simulink model "sensorFusionTask"  (R2015b)
settings: Solver=FixedStepDiscrete  StartTime=0.0  StopTime=inf  FixedStep=1/1000  RelTol=1e-3
libraries: simulink x3, embdlinuxlib x1
settings Model: SimulationMode=external  ExtModeEnableFloating=off  ExtModeTrigDuration=100  Creator=Nik Descher  LastModifiedBy=Nik Descher
settings DataIOCC: LimitDataPoints=off
settings OptimizationCC: OptimizeModelRefInitCode=on  LifeSpan=1
settings HardwareCC: ProdBitPerPointer=32  ProdLargestAtomicInteger=Long  ProdLargestAtomicFloat=Double  ProdWordSize=32  ProdHWDeviceType=ARM Compatible->ARM Cortex
settings RTWCC: SystemTargetFile=realtime.tlc  GenerateMakefile=off  TemplateMakefile=realtime.tmf  Description=Run on Target Hardware  RTWVerbose=off
settings STFCustomTargetCC: TargetLibSuffix=.a  GenerateSampleERTMain=on  ConcurrentExecutionCompliant=off  GeneratePreprocessorConditionals=Use local settings  ERTCustomFileBanners=on  SupportNonInlinedSFcns=off  SupportVariableSizeSignals=on  MATLABClassNameForMDSCustomization=Simulink.SoftwareTarget.ERTCustomization  CPPClassGenCompliant=off  GRTInterface=off  SystemTargetFile=realtime.tlc
settings ERTTargetCC: GenerateSampleERTMain=on  ParMdlRefBuildCompliant=off  CompOptLevelCompliant=off  ConcurrentExecutionCompliant=off  CombineOutputUpdateFcns=off  ERTFirstTimeCompliant=off  SupportContinuousTime=on  SupportVariableSizeSignals=on  ModelStepFunctionPrototypeControlCompliant=off  CPPClassGenCompliant=off  UseToolchainInfoCompliant=off  ExtModeMexArgs='192.168.1.248' 0 17724  ERTSrcFileBannerTemplate=realtime_code_template.cgt  ERTHdrFileBannerTemplate=realtime_code_template.cgt  ERTDataSrcFileTemplate=realtime_code_template.cgt  ERTDataHdrFileTemplate=realtime_code_template.cgt  ERTCustomFileTemplate=realtime_file_process.tlc

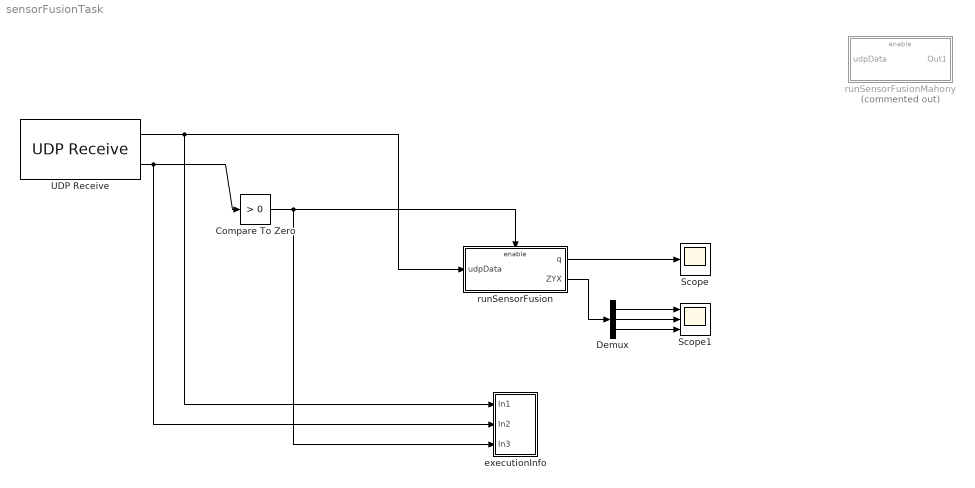
== system sensorFusionTask ==
  Compare To Zero : simulink/Logic and Bit Operations/Compare To Zero  relop=>  OutDataTypeStr=boolean
  Demux : Demux  Outputs=3
  Scope : Scope
  Scope1 : Scope  NumInputPorts=3
  UDP Receive : embdlinuxlib/UDP Receive  localURL='0.0.0.0'  localPort=25000  remoteURL='0.0.0.0'  remotePort=-1  recvBufferSize=8192  signalDatatype=single  dims=31  isVarSize=off  showBlockingTime=off  blockingTime=0  sampletime=1/1000  blockPlatform=Raspberry Pi
  executionInfo : Subsystem
  runSensorFusion : Subsystem  TreatAsAtomicUnit=on
  runSensorFusionMahony : Subsystem  Commented=on  TreatAsAtomicUnit=on
  wires:
  UDP Receive/1 -> executionInfo/1(In1), runSensorFusion/1(udpData)
  UDP Receive/2 -> executionInfo/2(In2), Compare To Zero/1
  Compare To Zero/1 -> executionInfo/3(In3), runSensorFusion/Enable
  runSensorFusion/1(q) -> Scope/1
  Demux/1 -> Scope1/1
  Demux/2 -> Scope1/2
  Demux/3 -> Scope1/3
  runSensorFusion/2(ZYX) -> Demux/1

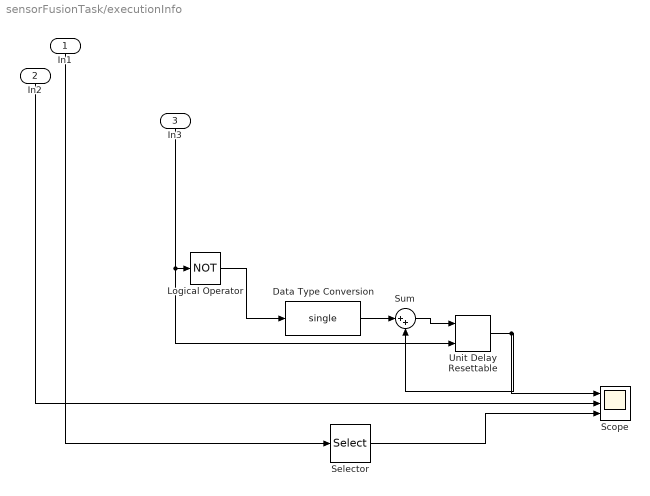
== system sensorFusionTask/executionInfo ==
  In1 : Inport
  In2 : Inport  Port=2
  In3 : Inport  Port=3
  Data Type Conversion : DataTypeConversion  OutDataTypeStr=single
  Logical Operator : Logic  Operator=NOT  AllPortsSameDT=off  OutDataTypeStr=boolean
  Scope : Scope  NumInputPorts=3
  Selector : Selector  InputPortWidth=31  IndexOptions=Index vector (dialog)  Indices=31  OutputSizes=1
  Sum : Sum  Inputs=|++
  Unit Delay Resettable : simulink/Additional Math & Discrete/Additional Discrete/Unit Delay Resettable  vinit=0  tsamp=-1
  wires:
  Unit Delay Resettable/1 -> Scope/1, Sum/2
  Data Type Conversion/1 -> Sum/1
  Sum/1 -> Unit Delay Resettable/1
  Logical Operator/1 -> Data Type Conversion/1
  Selector/1 -> Scope/3
  In3/1 -> Unit Delay Resettable/2, Logical Operator/1
  In1/1 -> Selector/1
  In2/1 -> Scope/2

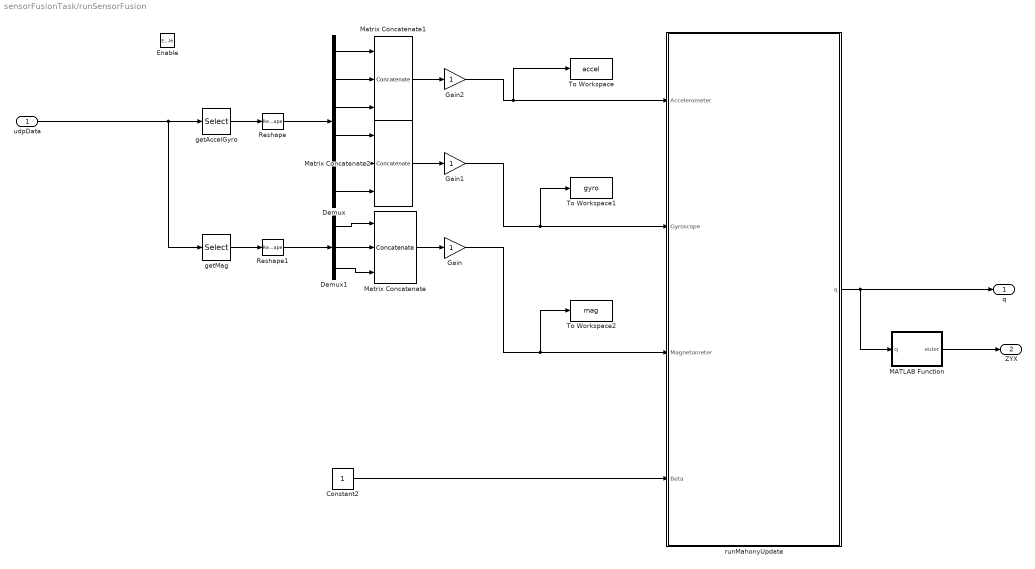
== system sensorFusionTask/runSensorFusion ==
  udpData : Inport
  Enable : EnablePort
  Constant2 : Constant  OutDataTypeStr=single
  Demux : Demux  Outputs=6
  Demux1 : Demux  Outputs=3
  Gain : Gain
  Gain1 : Gain
  Gain2 : Gain
  MATLAB Function : MATLAB Function  TreatAsAtomicUnit=on
  Matrix Concatenate : Concatenate  NumInputs=3  Mode=Multidimensional array
  Matrix Concatenate1 : Concatenate  NumInputs=3  Mode=Multidimensional array
  Matrix Concatenate2 : Concatenate  NumInputs=3  Mode=Multidimensional array
  Reshape : Reshape
  Reshape1 : Reshape
  To Workspace : ToWorkspace  VariableName=accel  SaveFormat=Structure With Time  SampleTime=-1
  To Workspace1 : ToWorkspace  VariableName=gyro  SaveFormat=Structure With Time  SampleTime=-1
  To Workspace2 : ToWorkspace  VariableName=mag  SaveFormat=Structure With Time  SampleTime=-1
  getAccelGyro : Selector  InputPortWidth=31  IndexOptions=Index vector (dialog)  Indices=1:24  OutputSizes=1
  getMag : Selector  InputPortWidth=31  IndexOptions=Index vector (dialog)  Indices=25:30  OutputSizes=1
  runMahonyUpdate : MATLAB Function  TreatAsAtomicUnit=on
  q : Outport
  ZYX : Outport  Port=2
  wires:
  getAccelGyro/1 -> Reshape/1
  Reshape/1 -> Demux/1
  Reshape1/1 -> Demux1/1
  udpData/1 -> getMag/1, getAccelGyro/1
  getMag/1 -> Reshape1/1
  Demux1/2 -> Matrix Concatenate/2
  Demux1/1 -> Matrix Concatenate/1
  Demux1/3 -> Matrix Concatenate/3
  Demux/2 -> Matrix Concatenate1/2
  Demux/3 -> Matrix Concatenate1/3
  Demux/1 -> Matrix Concatenate1/1
  Demux/4 -> Matrix Concatenate2/1
  Demux/5 -> Matrix Concatenate2/2
  Demux/6 -> Matrix Concatenate2/3
  Matrix Concatenate1/1 -> Gain2/1
  Matrix Concatenate2/1 -> Gain1/1
  Matrix Concatenate/1 -> Gain/1
  Constant2/1 -> runMahonyUpdate/4(Beta)
  runMahonyUpdate/1(q) -> MATLAB Function/1(q), q/1
  Gain/1 -> To Workspace2/1, runMahonyUpdate/3(Magnetometer)
  Gain1/1 -> To Workspace1/1, runMahonyUpdate/2(Gyroscope)
  Gain2/1 -> To Workspace/1, runMahonyUpdate/1(Accelerometer)
  MATLAB Function/1(euler) -> ZYX/1

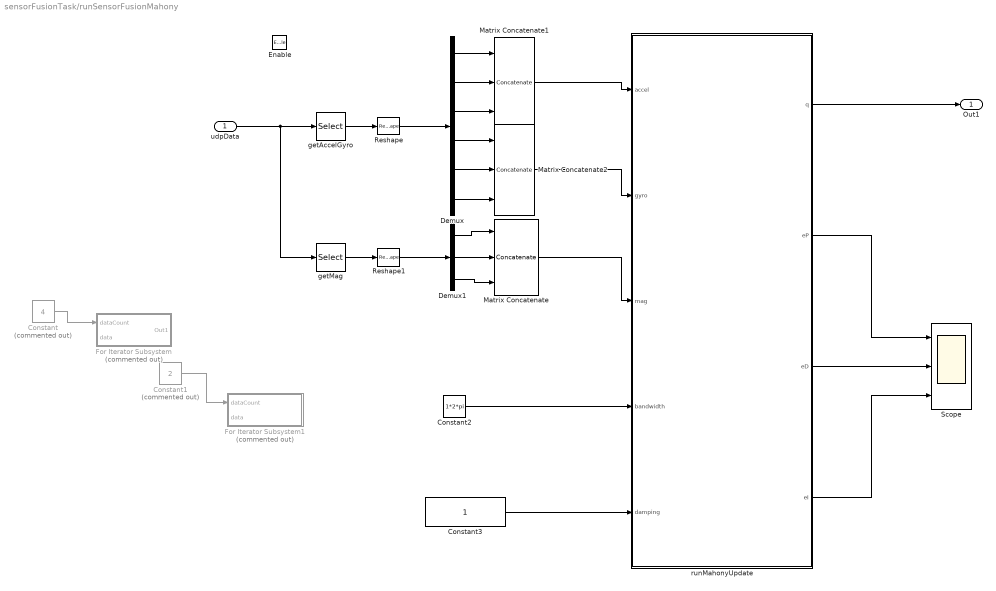
== system sensorFusionTask/runSensorFusionMahony ==
  udpData : Inport
  Enable : EnablePort
  Constant : Constant  Commented=on  Value=4
  Constant1 : Constant  Commented=on  Value=2
  Constant2 : Constant  Value=1*2*pi  OutDataTypeStr=single
  Constant3 : Constant  OutDataTypeStr=single
  Demux : Demux  Outputs=6
  Demux1 : Demux  Outputs=3
  For Iterator Subsystem : Subsystem  Commented=on  TreatAsAtomicUnit=on
  For Iterator Subsystem1 : Subsystem  Commented=on  TreatAsAtomicUnit=on
  Matrix Concatenate : Concatenate  NumInputs=3  Mode=Multidimensional array
  Matrix Concatenate1 : Concatenate  NumInputs=3  Mode=Multidimensional array
  Matrix Concatenate2 : Concatenate  NumInputs=3  Mode=Multidimensional array
  Reshape : Reshape
  Reshape1 : Reshape
  Scope : Scope  NumInputPorts=3
  getAccelGyro : Selector  InputPortWidth=31  IndexOptions=Index vector (dialog)  Indices=1:24  OutputSizes=1
  getMag : Selector  InputPortWidth=31  IndexOptions=Index vector (dialog)  Indices=25:30  OutputSizes=1
  runMahonyUpdate : MATLAB Function  TreatAsAtomicUnit=on
  Out1 : Outport
  wires:
  runMahonyUpdate/4(eI) -> Scope/3
  runMahonyUpdate/3(eD) -> Scope/2
  runMahonyUpdate/2(eP) -> Scope/1
  runMahonyUpdate/1(q) -> Out1/1
  Constant3/1 -> runMahonyUpdate/5(damping)
  Constant2/1 -> runMahonyUpdate/4(bandwidth)
  Matrix Concatenate/1 -> runMahonyUpdate/3(mag)
  Matrix Concatenate2/1 -> runMahonyUpdate/2(gyro)
  Matrix Concatenate1/1 -> runMahonyUpdate/1(accel)
  Demux/6 -> Matrix Concatenate2/3
  Demux/5 -> Matrix Concatenate2/2
  Demux/4 -> Matrix Concatenate2/1
  Demux/1 -> Matrix Concatenate1/1
  Demux/3 -> Matrix Concatenate1/3
  Demux/2 -> Matrix Concatenate1/2
  Demux1/3 -> Matrix Concatenate/3
  Demux1/1 -> Matrix Concatenate/1
  Demux1/2 -> Matrix Concatenate/2
  getMag/1 -> Reshape1/1
  udpData/1 -> getAccelGyro/1, getMag/1
  Reshape1/1 -> Demux1/1
  Reshape/1 -> Demux/1
  getAccelGyro/1 -> Reshape/1
  Constant1/1 -> For Iterator Subsystem1/1(dataCount)
  Constant/1 -> For Iterator Subsystem/1(dataCount)

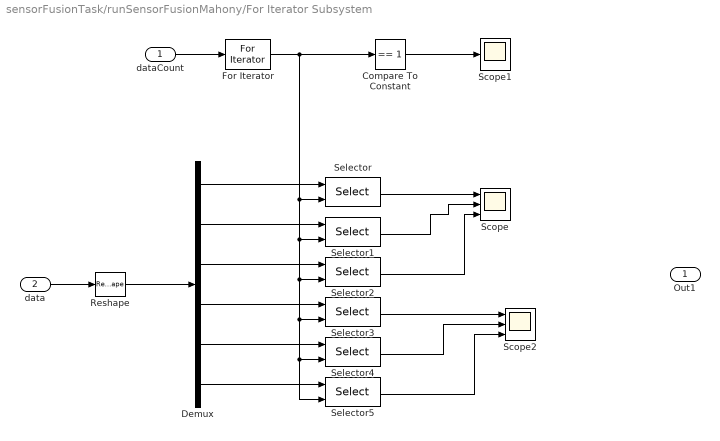
== system sensorFusionTask/runSensorFusionMahony/For Iterator Subsystem ==
  dataCount : Inport
  data : Inport  Port=2
  Compare To Constant : simulink/Logic and Bit Operations/Compare To Constant  relop===  const=1  OutDataTypeStr=boolean
  Demux : Demux  Outputs=6
  For Iterator : ForIterator  IterationSource=external
  Reshape : Reshape
  Scope : Scope  NumInputPorts=3
  Scope1 : Scope
  Scope2 : Scope  NumInputPorts=3
  Selector{,1..5} (6 alike) : Selector  InputPortWidth=4  IndexOptions=Index vector (port)  Indices=[1 3]  OutputSizes=1
  Out1 : Outport
  wires:
  Selector5/1 -> Scope2/3
  Selector4/1 -> Scope2/2
  Selector3/1 -> Scope2/1
  Reshape/1 -> Demux/1
  Compare To Constant/1 -> Scope1/1
  Selector2/1 -> Scope/3
  Selector1/1 -> Scope/2
  Selector/1 -> Scope/1
  Demux/6 -> Selector5/1
  Demux/5 -> Selector4/1
  Demux/4 -> Selector3/1
  Demux/3 -> Selector2/1
  Demux/2 -> Selector1/1
  For Iterator/1 -> Selector/2, Selector1/2, Selector2/2, Selector3/2, Selector4/2, Selector5/2, Compare To Constant/1
  Demux/1 -> Selector/1
  data/1 -> Reshape/1
  dataCount/1 -> For Iterator/1

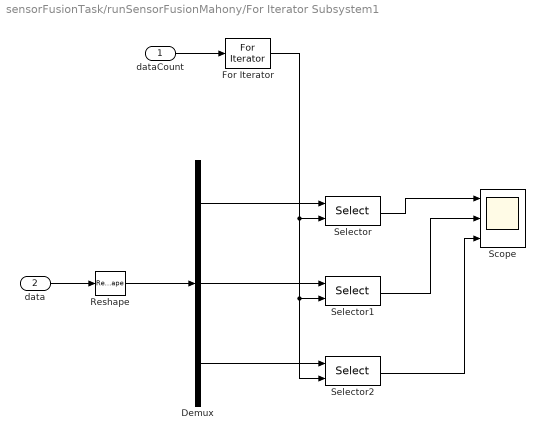
== system sensorFusionTask/runSensorFusionMahony/For Iterator Subsystem1 ==
  dataCount : Inport
  data : Inport  Port=2
  Demux : Demux  Outputs=3
  For Iterator : ForIterator  IterationSource=external
  Reshape : Reshape
  Scope : Scope  NumInputPorts=3
  Selector : Selector  InputPortWidth=2  IndexOptions=Index vector (port)  Indices=[1 3]  OutputSizes=1
  Selector1 : Selector  InputPortWidth=2  IndexOptions=Index vector (port)  Indices=[1 3]  OutputSizes=1
  Selector2 : Selector  InputPortWidth=2  IndexOptions=Index vector (port)  Indices=[1 3]  OutputSizes=1
  wires:
  dataCount/1 -> For Iterator/1
  data/1 -> Reshape/1
  Demux/1 -> Selector/1
  For Iterator/1 -> Selector2/2, Selector1/2, Selector/2
  Demux/2 -> Selector1/1
  Demux/3 -> Selector2/1
  Selector/1 -> Scope/1
  Selector1/1 -> Scope/2
  Selector2/1 -> Scope/3
  Reshape/1 -> Demux/1

== matlab function sensorFusionTask/runSensorFusionMahony/runMahonyUpdate ==
  data: accel input single size=[3 4]; q output; gyro input single size=[3 4]; mag input single size=[3 2]; bandwidth input; damping input; eP output; eD output; eI output
function [q,eP,eD,eI] = runMahonyUpdate(accel,gyro,mag,bandwidth,damping)
persistent qLocal
if isempty(qLocal)
    qLocal=single([ 1 0 0 0]);
end

magInterp=interp1([1 4],mag',[1 2 3 4],'linear')';

for i=1:4
    [qLocal,eP,eD,eI]=UpdateMahony(qLocal,gyro(:,i),accel(:,i),magInterp(:,i),bandwidth,damping);
end

q=qLocal;



 function [q,eP,eD,eI] = UpdateMahony(q,Gyroscope, Accelerometer, Magnetometer,bandwidth,damping)
     persistent eInt eLast
     if isempty(eInt)
         eInt=single([0; 0; 0]);
     end
     if abs(bandwidth)<1e-4 && abs(damping)<1e-4
         q=single([1 0 0 0]);
         eP=single([0;0;0]);
         eD=eP;
         eI=eP;
         return;
     end
%      bandwidth = (1*2*pi);
%      damping=1;
     Ki=bandwidth^2*bandwidth;
     Kp=bandwidth^2+2*damping*bandwidth*bandwidth;
     Kd=2*damping*bandwidth+bandwidth;
% 
%      Ki=0;
%      Kp=1;
%      Kd=0;
     
     SamplePeriod=5/1000;
     % Normalise accelerometer measurement
%      if(norm(Accelerometer) == 0), return; end   % handle NaN
     Accelerometer = Accelerometer / norm(Accelerometer);    % normalise magnitude
     
     % Normalise magnetometer measurement
%      if(norm(Magnetometer) == 0), return; end    % handle NaN
     Magnetometer = Magnetometer / norm(Magnetometer);   % normalise magnitude
     
     % Reference direction of Earth's magnetic feild
     h = quaternProd(q, quaternProd([0; Magnetometer], quaternConj(q)));
     b = [0; norm([h(2); h(3)]); 0; h(4)];
     
     % Estimated direction of gravity and magnetic field
     v = [2*(q(2)*q(4) - q(1)*q(3))
         2*(q(1)*q(2) + q(3)*q(4))
         q(1)^2 - q(2)^2 - q(3)^2 + q(4)^2];
     w = [2*b(2)*(0.5 - q(3)^2 - q(4)^2) + 2*b(4)*(q(2)*q(4) - q(1)*q(3))
         2*b(2)*(q(2)*q(3) - q(1)*q(4)) + 2*b(4)*(q(1)*q(2) + q(3)*q(4))
         2*b(2)*(q(1)*q(3) + q(2)*q(4)) + 2*b(4)*(0.5 - q(2)^2 - q(3)^2)];
     
     % Error is sum of cross product between estimated direction and measured direction of fields
     e = cross(Accelerometer, v) + cross(Magnetometer, w);
     if(Ki > 0)
         eInt = eInt + e * SamplePeriod;
     else
         eInt = single([0; 0; 0]);
     end
     if isempty(eLast)
         eLast=e;
     end
     
     % Apply feedback terms
     eP=e;
     eD=e-eLast;
     eI=eInt;
     Gyroscope = Gyroscope + Kp * eP + Ki * eInt + Kd * (eD) / SamplePeriod;
     eLast=e;
     
     % Compute rate of change of quaternion
     qDot = 0.5 * quaternProd(q, [0 Gyroscope(1) Gyroscope(2) Gyroscope(3)]);
     
     % Integrate to yield quaternion
     q = q + qDot * SamplePeriod;
     q = q / norm(q); % normalise quaternion
     

function ab = quaternProd(a, b)
    ab=zeros(1,4);
%QUATERNPROD Calculates the quaternion product
%
%   ab = quaternProd(a, b)
%
%   Calculates the quaternion product of quaternion a and b.
%
%   For more information see:
%   http://www.x-io.co.uk/node/8#quaternions
%
%	Date          Author          Notes
%	27/09/2011    SOH Madgwick    Initial release

    ab(1) = a(1).*b(1)-a(2).*b(2)-a(3).*b(3)-a(4).*b(4);
    ab(2) = a(1).*b(2)+a(2).*b(1)+a(3).*b(4)-a(4).*b(3);
    ab(3) = a(1).*b(3)-a(2).*b(4)+a(3).*b(1)+a(4).*b(2);
    ab(4) = a(1).*b(4)+a(2).*b(3)-a(3).*b(2)+a(4).*b(1);

function qConj = quaternConj(q)
%QUATERN2ROTMAT Converts a quaternion to its conjugate
%
%   qConj = quaternConj(q)
%
%   Converts a quaternion to its conjugate.
%
%   For more information see:
%   http://www.x-io.co.uk/node/8#quaternions
%
%	Date          Author          Notes
%	27/09/2011    SOH Madgwick    Initial release

    qConj = [q(1) -q(2) -q(3) -q(4)];

== matlab function sensorFusionTask/runSensorFusion/runMahonyUpdate ==
  data: Accelerometer input single size=[3 4]; q output single size=[1 4]; Gyroscope input single size=[3 4]; Magnetometer input single size=[3 2]; Beta input single size=1
function q  = runMadwickUpdates(Accelerometer,Gyroscope,Magnetometer,Beta)
persistent qLocal
if isempty(qLocal)
    qLocal=single([1 0 0 0]);
end
qIn=qLocal;

magInterp=interp1([1 4],Magnetometer',[1 2 3 4],'linear')';

for i=1:4
    
    q  = runMadwickUpdate(qIn,Accelerometer(:,i),Gyroscope(:,i),magInterp(:,i),Beta);
    qIn = q;
    
end

qLocal=q;

function q  = runMadwickUpdate(qIn,Accelerometer,Gyroscope,Magnetometer,Beta)
q=qIn;
SamplePeriod=single(5/1000);

% Normalise accelerometer measurement
if ~all(abs(Accelerometer)<.0001);
    Accelerometer = Accelerometer / norm(Accelerometer);	% normalise magnitude
end
% Normalise magnetometer measurement
if ~all(abs(Magnetometer)<.0001)
    Magnetometer = Magnetometer / norm(Magnetometer);	% normalise magnitude
end
% Reference direction of Earth's magnetic feild
h = quaternProd(q, quaternProd([0 Magnetometer'], quaternConj(q)));
b = [0 norm([h(2) h(3)]) 0 h(4)];
% Gradient decent algorithm corrective step
F = [2*(q(2)*q(4) - q(1)*q(3)) - Accelerometer(1)
    2*(q(1)*q(2) + q(3)*q(4)) - Accelerometer(2)
    2*(0.5 - q(2)^2 - q(3)^2) - Accelerometer(3)
    2*b(2)*(0.5 - q(3)^2 - q(4)^2) + 2*b(4)*(q(2)*q(4) - q(1)*q(3)) - Magnetometer(1)
    2*b(2)*(q(2)*q(3) - q(1)*q(4)) + 2*b(4)*(q(1)*q(2) + q(3)*q(4)) - Magnetometer(2)
    2*b(2)*(q(1)*q(3) + q(2)*q(4)) + 2*b(4)*(0.5 - q(2)^2 - q(3)^2) - Magnetometer(3)];
J = [-2*q(3),                 	2*q(4),                    -2*q(1),                         2*q(2)
    2*q(2),                 	2*q(1),                    	2*q(4),                         2*q(3)
    0,                         -4*q(2),                    -4*q(3),                         0
    -2*b(4)*q(3),               2*b(4)*q(4),               -4*b(2)*q(3)-2*b(4)*q(1),       -4*b(2)*q(4)+2*b(4)*q(2)
    -2*b(2)*q(4)+2*b(4)*q(2),	2*b(2)*q(3)+2*b(4)*q(1),	2*b(2)*q(2)+2*b(4)*q(4),       -2*b(2)*q(1)+2*b(4)*q(3)
    2*b(2)*q(3),                2*b(2)*q(4)-4*b(4)*q(2),	2*b(2)*q(1)-4*b(4)*q(3),        2*b(2)*q(2)];
step = (J'*F);
step = step / norm(step);	% normalise step magnitude

% Compute rate of change of quaternion
qDot = 0.5 * quaternProd(q, [0 Gyroscope(1) Gyroscope(2) Gyroscope(3)]) - Beta * step';

% Integrate to yield quaternion
q = q + qDot * SamplePeriod;
q = q / norm(q); % normalise quaternion


function ab = quaternProd(a, b)
    ab=zeros(1,4);
%QUATERNPROD Calculates the quaternion product
%
%   ab = quaternProd(a, b)
%
%   Calculates the quaternion product of quaternion a and b.
%
%   For more information see:
%   http://www.x-io.co.uk/node/8#quaternions
%
%	Date          Author          Notes
%	27/09/2011    SOH Madgwick    Initial release

    ab(1) = a(1).*b(1)-a(2).*b(2)-a(3).*b(3)-a(4).*b(4);
    ab(2) = a(1).*b(2)+a(2).*b(1)+a(3).*b(4)-a(4).*b(3);
    ab(3) = a(1).*b(3)-a(2).*b(4)+a(3).*b(1)+a(4).*b(2);
    ab(4) = a(1).*b(4)+a(2).*b(3)-a(3).*b(2)+a(4).*b(1);

function qConj = quaternConj(q)
%QUATERN2ROTMAT Converts a quaternion to its conjugate
%
%   qConj = quaternConj(q)
%
%   Converts a quaternion to its conjugate.
%
%   For more information see:
%   http://www.x-io.co.uk/node/8#quaternions
%
%	Date          Author          Notes
%	27/09/2011    SOH Madgwick    Initial release

    qConj = [q(1) -q(2) -q(3) -q(4)];

== matlab function sensorFusionTask/runSensorFusion/MATLAB Function ==
  data: q input single size=4; euler output single size=[1 3]
function euler = quatern2euler(q)
%#codegen

%QUATERN2EULER Converts a quaternion orientation to ZYX Euler angles
%
%   q = quatern2euler(q)
%
%   Converts a quaternion orientation to ZYX Euler angles where phi is a
%   rotation around X, theta around Y and psi around Z.
%
%   For more information see:
%   http://www.x-io.co.uk/node/8#quaternions
%
%	Date          Author          Notes
%	27/09/2011    SOH Madgwick    Initial release
R=zeros(3,'single');
    R(1,1) = 2.*q(1).^2-1+2.*q(2).^2;
    R(2,1) = 2.*(q(2).*q(3)-q(1).*q(4));
    R(3,1) = 2.*(q(2).*q(4)+q(1).*q(3));
    R(3,2) = 2.*(q(3).*q(4)-q(1).*q(2));
    R(3,3) = 2.*q(1).^2-1+2.*q(4).^2;

    phi = atan2(R(3,2), R(3,3) );
    theta = -atan(R(3,1) ./ sqrt(1-R(3,1).^2) );
    psi = atan2(R(2,1), R(1,1) );

    euler = [phi(1)' theta(1)' psi(1)'];
end
